simulink model "digital_com_3rd_lab"  (R2022b)
settings: Solver=VariableStepAuto  StartTime=0.0  StopTime=0.1  RelTol=1e-3
libraries: simulink x1, dspsigops x1, dspquant2 x1
settings Model: Creator=Asus  LastModifiedBy=Asus

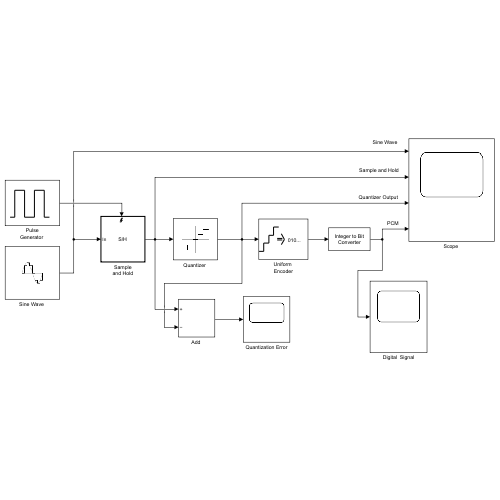
[thumbnail: Simulink's stored preview of the top-level diagram]
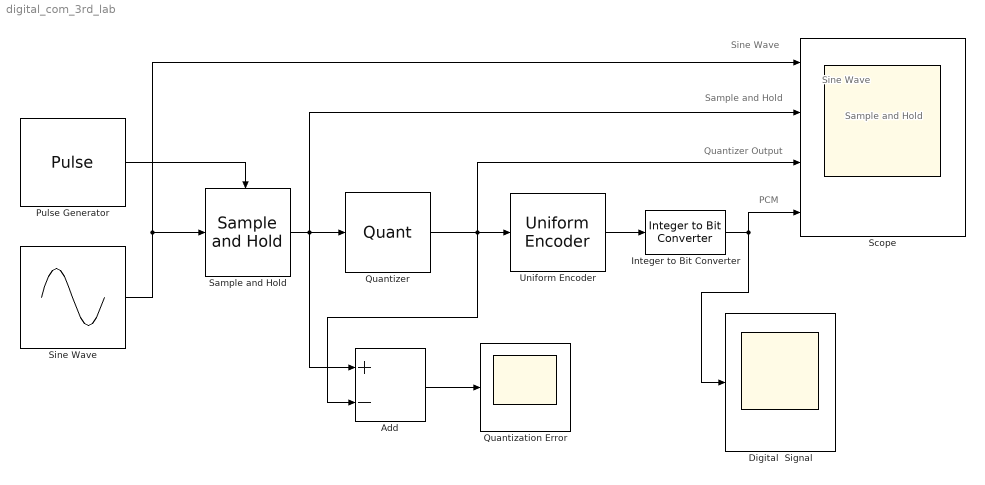
== system digital_com_3rd_lab ==
  note: Sine Wave
  note: Sample
      | and Hold
  note: Sine Wave
  note: Sample and Hold
  note: PCM
  note: Quantizer Output
  "Add " : Sum  Inputs=+-
  Digital  Signal : Scope
  Integer to Bit Converter : simulink/Logic and Bit Operations/Integer to Bit Converter  nbits=8  signedInputValues=Unsigned  bitOrder=MSB first  outDtype=Inherit via internal rule
  "Pulse Generator " : DiscretePulseGenerator  PulseType=Time based  Period=1/3000  PulseWidth=30
  Quantization Error : Scope
  "Quantizer " : Quantizer  QuantizationInterval=1  LinearizeAsGain=off
  Sample and Hold : dspsigops/Sample and Hold  trig=Rising edge  initCond=0  latchinput=off
  "Scope " : Scope  NumInputPorts=4
  "Sine Wave " : Sin  Amplitude=5  Frequency=2*pi*50  SampleTime=1/50000
  Uniform Encoder : dspquant2/Uniform Encoder  peak=5  bits=8  otype=Unsigned integer
  wires:
  "Pulse Generator "/1 -> Sample and Hold/Trigger
  "Sine Wave "/1 -> "Scope "/1, Sample and Hold/1
  Sample and Hold/1 -> "Quantizer "/1, "Scope "/2, "Add "/1
  "Quantizer "/1 -> "Add "/2, "Scope "/3, Uniform Encoder/1
  Uniform Encoder/1 -> Integer to Bit Converter/1
  Integer to Bit Converter/1 -> Digital  Signal/1, "Scope "/4
  "Add "/1 -> Quantization Error/1
